simulink model "bassengmodell_1"  (R2014b)
settings: Solver=ode45  StartTime=0.0  StopTime=10  FixedStep=0.1  RelTol=1e-3
values from neighbouring files (symbols this model uses):
  A = V/300    (= 378541.178)    [main_1.m]    (also in main_rev2.m = 10)
  C_pv = 4.1796    [main_1.m]    (also in main_rev2.m)
  h = 5.7 + 3.8*vind    (= 24.7)    [main_1.m]    (also in main_rev2.m = 2)
  T_0 = 15+273.15    (= 288.15)    [main_1.m]    (also in main_rev2.m = 15)
  T_om = 15+273.15    (= 288.15)    [main_1.m]    (also in main_rev2.m = 15)
  T_onsket = 30+273.15    (= 303.15)    [main_1.m]    (also in main_rev2.m = 30)
  V = 30000*3785.41178    (= 113562353.4)    [main_1.m]    (also in main_rev2.m = 20000000)
libraries: simulink x1
settings Model: Creator=rende_000  LastModifiedBy=rende_000

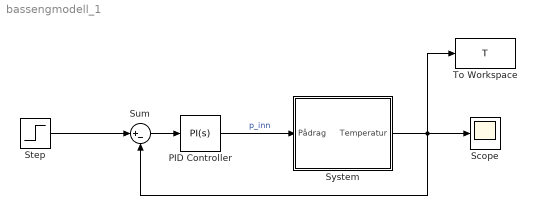
== system bassengmodell_1 ==
  PID Controller : simulink/Continuous/PID Controller  Controller=PI  TimeDomain=Continuous-time  SampleTime=-1  IntegratorMethod=Forward Euler  FilterMethod=Forward Euler  Form=Parallel  P=300000000  I=0  D=0  N=100  InitialConditionSource=internal  InitialConditionForIntegrator=0  InitialConditionForFilter=0  ExternalReset=none  LimitOutput=off  UpperSaturationLimit=inf  LowerSaturationLimit=-inf  LinearizeAsGain=on  AntiWindupMode=none  Kb=1  TrackingMode=off  Kt=1  PParamMin=[]  PParamMax=[]  IParamMin=[]  IParamMax=[]  DParamMin=[]  DParamMax=[]  NParamMin=[]  NParamMax=[]  KbParamMin=[]  KbParamMax=[]  KtParamMin=[]  KtParamMax=[]  POutMin=[]  POutMax=[]  IOutMin=[]  IOutMax=[]  DOutMin=[]  DOutMax=[]  NOutMin=[]  NOutMax=[]  KbOutMin=[]  KbOutMax=[]  KtOutMin=[]  KtOutMax=[]  IntegratorOutMin=[]  IntegratorOutMax=[]  FilterOutMin=[]  FilterOutMax=[]  SumOutMin=[]  SumOutMax=[]  SumI1OutMin=[]  SumI1OutMax=[]  SumI2OutMin=[]  SumI2OutMax=[]  SumI3OutMin=[]  SumI3OutMax=[]  SumDOutMin=[]  SumDOutMax=[]  SaturationOutMin=[]  SaturationOutMax=[]  IntegratorContinuousStateAttributes=''  IntegratorStateMustResolveToSignalObject=off  IntegratorRTWStateStorageClass=Auto  FilterContinuousStateAttributes=''  FilterStateMustResolveToSignalObject=off  FilterRTWStateStorageClass=Auto  DifferentiatorICPrevScaledInput=0  DifferentiatorOutMin=[]  DifferentiatorOutMax=[]  UseFilter=on
  Scope : Scope
  Step : Step  Time=10000  Before=T_om  After=T_onsket  SampleTime=0
  Sum : Sum  Inputs=|+-
  System : Subsystem
  To Workspace : ToWorkspace  VariableName=T  SaveFormat=Timeseries  SampleTime=-1
  wires:
  PID Controller/1 -> System/1(Pådrag)  "p_inn"
  Sum/1 -> PID Controller/1
  System/1(Temperatur) -> Sum/2, Scope/1, To Workspace/1
  Step/1 -> Sum/1

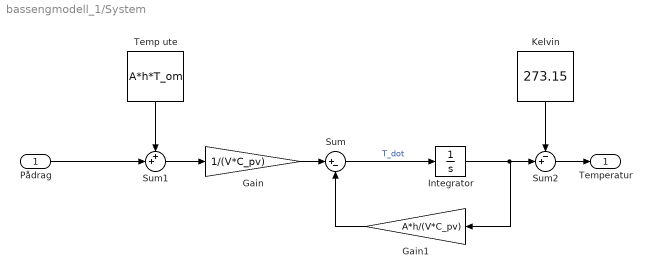
== system bassengmodell_1/System ==
  Pådrag : Inport
  Gain : Gain  Gain=1/(V*C_pv)
  Gain1 : Gain  Gain=A*h/(V*C_pv)
  Integrator : Integrator  InitialCondition=T_0
  Kelvin : Constant  Value=273.15
  Sum : Sum  Inputs=|+-
  Sum1 : Sum  Inputs=++|
  Sum2 : Sum  Inputs=-+|
  Temp ute : Constant  Value=A*h*T_om
  Temperatur : Outport
  wires:
  Integrator/1 -> Sum2/2, Gain1/1
  Sum/1 -> Integrator/1  "T_dot"
  Gain/1 -> Sum/1
  Temp ute/1 -> Sum1/1
  Gain1/1 -> Sum/2
  Sum1/1 -> Gain/1
  Pådrag/1 -> Sum1/2
  Kelvin/1 -> Sum2/1
  Sum2/1 -> Temperatur/1
